simulink model "NEDI"  (R2023a)
settings: Solver=FixedStepDiscrete  StartTime=0.0  StopTime=simTime  RelTol=1e-3
InitFcn:
  | % block settings for 240p, change format as appropriate
  | frm2pix = visionhdl.FrameToPixels;
  | frm2pix.VideoFormat = '240p';
  | [activePixelsPerLine, activeLines, totalPixels] = getparamfromfrm2pix(frm2pix);
  | numFrames = 10;
  | simTime = totalPixels * numFrames;
  | % pixel control bus
  | evalin('base','pixelcontrolbus');
values from neighbouring files (symbols this model uses):
  C = double(zeros(m^2, 4))    [NEDI.m]
undefined symbols (not defined in the file or in its folder): gray, none, videoinput
libraries: imaqlib x1
settings Model: DataTypeOverride=Off  SimulationMode=accelerator  Creator=14689  LastModifiedBy=14689
settings SolverCC: AlgebraicLoopSolver=TrustRegion  AutoInsertRateTranBlk=on  MaxZcPerStep=1
settings DataIOCC: LimitDataPoints=on  SaveOutput=off  SaveTime=off
settings OptimizationCC: BlockReduction=off  ConditionallyExecuteInputs=off  DefaultParameterBehavior=Inlined  LifeSpan=inf
settings DebuggingCC: AlgebraicLoopMsg=error  SingleTaskRateTransMsg=error  UnconnectedInputMsg=warning  UnconnectedOutputMsg=warning  UnconnectedLineMsg=warning  AllowSymbolicDim=off  SubsystemReferenceDiagnosticForUnitTest=warning  StrictBusMsg=ErrorOnBusTreatedAsVector  SFUnexpectedBacktrackingDiag=warning  SFNoUnconditionalDefaultTransitionDiag=warning  SFExecutionAtInitializationDiag=none  ArithmeticOperatorsInVariantConditions=warning
settings HardwareCC: ProdBitPerPointer=32  ProdBitPerSizeT=32  ProdBitPerPtrDiffT=32  ProdLargestAtomicFloat=None  ProdIntDivRoundTo=Undefined  ProdEndianess=Unspecified  ProdWordSize=32  ProdHWDeviceType=ASIC/FPGA->ASIC/FPGA  TargetBitPerPointer=64  TargetBitPerSizeT=64  TargetBitPerPtrDiffT=64  TargetLongLongMode=on  TargetIntDivRoundTo=Zero  TargetEndianess=LittleEndian  TargetWordSize=64  TargetHWDeviceType=Custom Processor->MATLAB Host Computer  ProdEqTarget=off
settings ModelReferenceCC: EnableRefExpFcnMdlSchedulingChecks=on
settings SFSimCC: SimUseLocalCustomCode=off  CustomCodeUndefinedFunction=UseInterfaceOnly
settings RTWCC: RTWUseLocalCustomCode=off  DLArmComputeVersion=19.05
settings CodeAppCC: StateflowObjectComments=on
settings GRTTargetCC: TargetLangStandard=C89/C90 (ANSI)
settings ConfigComp: CovMetricSettings=dw  CovSaveCumulativeToWorkspaceVar=on  CovSaveSingleToWorkspaceVar=on  CovExternalEMLEnable=off  CovSFcnEnable=off

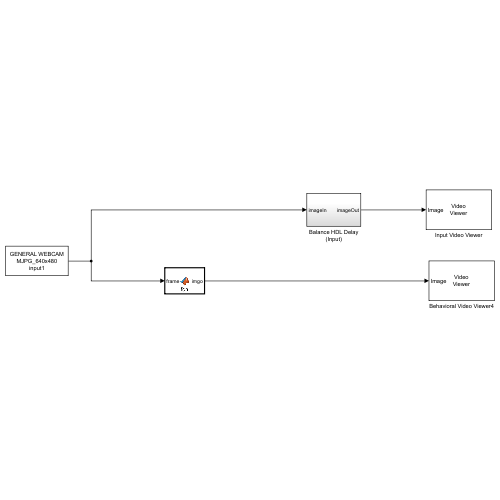
[thumbnail: Simulink's stored preview of the top-level diagram]
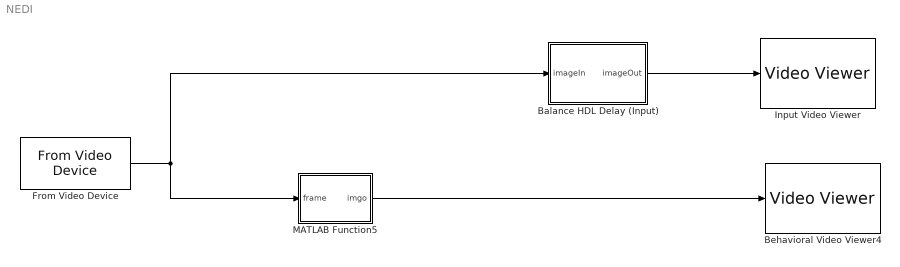
== system NEDI ==
  Balance HDL Delay (Input) : Subsystem
  Behavioral Video Viewer4 : VideoViewer  colormapValue=gray(256)  FigPos=[3525 1092.66666666667 957.333333333333 926]
  From Video Device : imaqlib/From Video Device  DeviceMenu=(none)  Device=winvideo 1 (GENERAL WEBCAM)  ObjConstructor=videoinput('winvideo', 1)  VideoFormatMenu=(none)  VideoFormat=MJPG_640x480  VideoSource=input1  ROIPosition=[0 0 480 640]  EnableHWTrigger=off  TriggerConfiguration=none/none  SampleTime=1/30  OutputPortsMode=One multidimensional signal  DataType=double  CanDoHWTrigger=no  ReturnedColorSpace=rgb  BlockHandle=1647.0001  ROIWidth=640  ROIHeight=480  ROIColumn=0  ROIRow=0  EngXMLPath=C:\Program Files\MATLAB\R2023a\toolbox\imaq\imaq\private  DevXMLPath=C:\ProgramData\MATLAB\SupportPackages\R2023a\toolbox\imaq\supportpackages\genericvideo\adaptor\win64  EngLibPath=C:\Program Files\MATLAB\R2023a\toolbox\imaq\imaqblks\imaqmex\win64  ColorSpace=rgb  BayerSensorAlignment=grbg  ImaqMode=off
  Input Video Viewer : VideoViewer  colormapValue=gray(256)  FigPos=[2563.66666666667 1078.66666666667 957.333333333333 926]
  MATLAB Function5 : MATLAB Function  TreatAsAtomicUnit=on
  wires:
  Balance HDL Delay (Input)/1(imageOut) -> Input Video Viewer/1
  From Video Device/1 -> MATLAB Function5/1(frame), Balance HDL Delay (Input)/1(imageIn)
  MATLAB Function5/1(imgo) -> Behavioral Video Viewer4/1

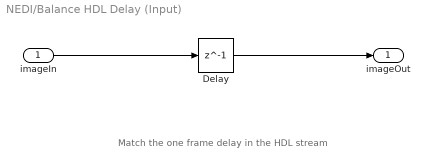
== system NEDI/Balance HDL Delay (Input) ==
  note: Match the one frame delay in the HDL stream
  imageIn : Inport
  Delay : Delay  DelayLength=1
  imageOut : Outport
  wires:
  imageIn/1 -> Delay/1
  Delay/1 -> imageOut/1

== matlab function NEDI/MATLAB Function5 ==
  data: frame input; imgo output
function imgo = fcn(frame)

m = 5; % window size
s = 2; % scale size

dims = size(frame);
rows = dims(1);
cols = dims(2);
targetSize = [2*rows, 2*cols];


% Canny edge detection
img=im2double(frame);

I=rgb2gray(img);

sharp = edge(I,'canny', 0.3);


% insert low-resolution pixels
imgo = imresize(img, targetSize, 'bicubic');


y = double(zeros(m^2, 1)); % pixels in the window
C = double(zeros(m^2, 4)); % interpolation neighbours of each pixel in the window


%% step 1  reconstruct the points with the form of (2*i+1,2*j+1)
for k=1:3  % 3 colors
    for i=4:rows-4
        for j=4:cols-4
                if(sharp(i,j)==1)
                temp=1;
                for ii=(i+1-ceil(m/2)):(i+floor(m/2))
                   for jj=j+1-ceil(m/2):j+floor(m/2)
                       y(temp)=imgo(2*ii,2*jj,k);
                       C(temp,1)=imgo(2*ii-2,2*jj-2,k);
                       C(temp,2)=imgo(2*ii+2,2*jj-2,k);
                       C(temp,3)=imgo(2*ii+2,2*jj+2,k);
                       C(temp,4)=imgo(2*ii-2,2*jj+2,k);
                       temp=temp+1;                     
                   end
                end
                alpha = pinv(C' * C) * C' * y;
                imgo(2*i+1,2*j+1,k)=(alpha(1)*imgo(2*i,2*j,k)+alpha(2)*imgo(2*i+2,2*j,k)...
                    +alpha(3)*imgo(2*i+2,2*j+2,k)+alpha(4)*imgo(2*i,2*j+2,k));
                    
            end
        end
    end 
end


%% step 2 reconstructed the points with the forms of (2*i+1,2*j)
for k=1:3  % 3 colors
    for i=4:rows-4
        for j=4:cols-4
                if(sharp(i,j)==1)
                temp=1;
                for ii=(i+1-ceil(m/2)):(i+floor(m/2))
                   for jj=j+1-ceil(m/2):j+floor(m/2)
                       y(temp)=imgo(2*ii+1,2*jj-1,k);
                       C(temp,1)=imgo(2*ii-1,2*jj-1,k);
                       C(temp,2)=imgo(2*ii+1,2*jj-3,k);
                       C(temp,3)=imgo(2*ii+3,2*jj-1,k);
                       C(temp,4)=imgo(2*ii+1,2*jj+1,k);
                       temp=temp+1;                     
                   end
                end
                alpha = pinv(C' * C) * C' * y;
                imgo(2*i+1,2*j,k)=(alpha(1)*imgo(2*i,2*j,k)+alpha(2)*imgo(2*i+1,2*j-1,k)...
                    +alpha(3)*imgo(2*i+2,2*j,k)+alpha(4)*imgo(2*i+1,2*j+1,k));
            end
        end
    end  
end

%% step 3 reconstructed the points with the forms of (2*i,2*j+1)

for k=1:3  % 3 colors
    for i=4:rows-4
        for j=4:cols-4
                if(sharp(i,j)==1)
                temp=1;
                for ii=(i+1-ceil(m/2)):(i+floor(m/2))
                   for jj=j+1-ceil(m/2):j+floor(m/2)
                       y(temp)=imgo(2*ii+1,2*jj-1,k);
                       C(temp,1)=imgo(2*ii-1,2*jj-1,k);
                       C(temp,2)=imgo(2*ii+1,2*jj-3,k);
                       C(temp,3)=imgo(2*ii+3,2*jj-1,k);
                       C(temp,4)=imgo(2*ii+1,2*jj+1,k);
                       temp=temp+1;                     
                   end
                end
                alpha = pinv(C' * C) * C' * y;
                imgo(2*i,2*j+1,k)=(alpha(1)*imgo(2*i-1,2*j+1,k)+alpha(2)*imgo(2*i,2*j,k)...
                    +alpha(3)*imgo(2*i+1,2*j+1,k)+alpha(4)*imgo(2*i,2*j+2,k));
            end
        end
    end  
end
